simulink model "Prob2"  (R2017b)
settings: Solver=ode4  StartTime=0.0  StopTime=10.0  FixedStep=0.1  RelTol=1e-3
values from neighbouring files (symbols this model uses):
  den = [0.3739 1.3343 0.5280 0.0381  -0.0235]    [Problem3.m]    (also in Problem4.m = [0.0475 0.05 0.735]; Problem5.m = [1 0.039 0.053]; Run_Prob2.m = [0.1539*(Lv/u0)^3 1.9754*(Lv/u0)^2 2.9958*(Lv/u0) 1])
  num = [0.25*Kp]    [Problem4.m]    (also in Problem5.m = [0.038 0]; Run_Prob2.m = alv*sqrt(Lv/u0)*[0.3398*(Lv/u0)^2 2.7478*(Lv/u0) 1])
  x0 = [0;0;0;0]    [Run_Prob2.m]
libraries: simulink x1, simulink_extras x1
settings Model: Creator=Daslab  LastModifiedBy=Daslab

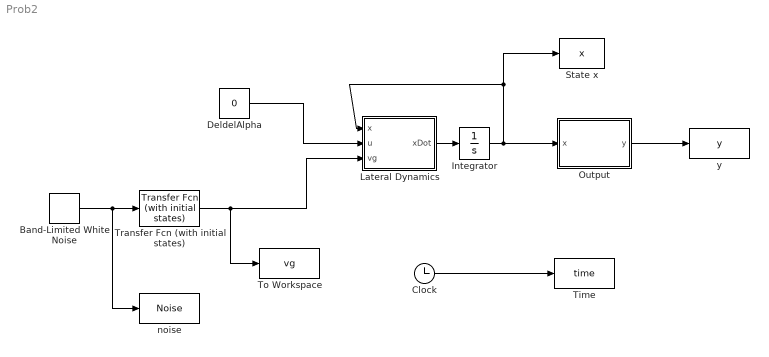
== system Prob2 ==
  "Band-Limited White Noise " : simulink/Sources/Band-Limited White Noise  Cov=[0.1]  Ts=0.1  seed=[25533]
  Clock : Clock
  DeldelAlpha : Constant  Value=0
  Integrator : Integrator  InitialCondition=x0
  Lateral Dynamics : MATLAB Function  TreatAsAtomicUnit=on
  "Output " : MATLAB Function  TreatAsAtomicUnit=on
  "State x " : ToWorkspace  VariableName=x  SampleTime=-1
      settings: Save2DSignal=2-D array (concatenate along first dimension)
  "Time " : ToWorkspace  VariableName=time  SampleTime=-1
      settings: Save2DSignal=2-D array (concatenate along first dimension)
  "To Workspace " : ToWorkspace  VariableName=vg  SampleTime=-1
      settings: Save2DSignal=2-D array (concatenate along first dimension)
  "Transfer Fcn (with initial states) " : simulink_extras/Additional Linear/Transfer Fcn (with initial states)  N=num  D=den  X0=0
  "noise " : ToWorkspace  VariableName=Noise  SampleTime=-1
      settings: Save2DSignal=2-D array (concatenate along first dimension)
  "y " : ToWorkspace  VariableName=y  SampleTime=-1
      settings: Save2DSignal=2-D array (concatenate along first dimension)
  wires:
  Lateral Dynamics/1(xDot) -> Integrator/1
  Integrator/1 -> "State x "/1, Lateral Dynamics/1(x), "Output "/1(x)
  DeldelAlpha/1 -> Lateral Dynamics/2(u)
  "Output "/1(y) -> "y "/1
  "Band-Limited White Noise "/1 -> "noise "/1, "Transfer Fcn (with initial states) "/1
  "Transfer Fcn (with initial states) "/1 -> "To Workspace "/1, Lateral Dynamics/3(vg)
  Clock/1 -> "Time "/1

== matlab function Prob2/Output  ==
  data: x input; y output
function y = fcn(x)

u0 = 272; % m/s 
C = [-0.5*u0 0 0 0];

y = C*x;

== matlab function Prob2/Lateral Dynamics ==
  data: x input; u input; xDot output; vg input
function xDot = fcn(x,u,vg)

A = [-0.5,  0, -1, 0.02;
     -150, -7, -0.15, 0;
     30, 0.1, -1, 0; 
     0 1 0 0]; 
 
B = [-0.02, 56, 1, 0]';

G = [0.5; 150; -30; 0];  

xDot = A*x+ B*u + G*vg;
